simulink model "FINAL100225conmatlab2021"  (R2023a)
settings: Solver=VariableStepAuto  StartTime=0.0  StopTime=100  RelTol=1e-3
libraries: cstblocks x1
settings Model: Creator=cgbri  LastModifiedBy=Maxi
settings RTWCC: GPUComputeCapability=5.0

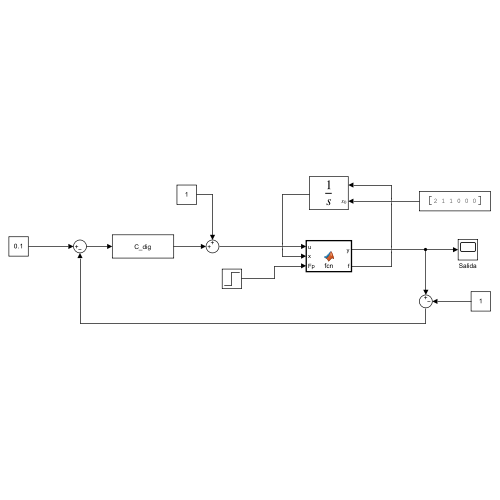
[thumbnail: Simulink's stored preview of the top-level diagram]
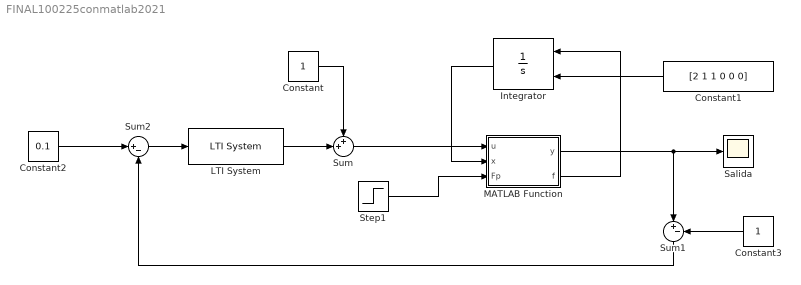
== system FINAL100225conmatlab2021 ==
  Constant : Constant
  Constant1 : Constant  Value=[2 1 1 0 0 0]
  Constant2 : Constant  Value=0.1
  Constant3 : Constant
  Integrator : Integrator  InitialConditionSource=external
  LTI System : cstblocks/LTI System  sys=C_dig  IC=[]
  MATLAB Function : MATLAB Function  TreatAsAtomicUnit=on
  Salida : Scope
  Step1 : Step  After=0  SampleTime=0
  Sum : Sum  Inputs=++|
  Sum1 : Sum  Inputs=|+-
  Sum2 : Sum  Inputs=|+-
  wires:
  Integrator/1 -> MATLAB Function/2(x)
  MATLAB Function/2(f) -> Integrator/1
  Constant1/1 -> Integrator/2
  Step1/1 -> MATLAB Function/3(Fp)
  MATLAB Function/1(y) -> Sum1/1, Salida/1
  Sum/1 -> MATLAB Function/1(u)
  Constant/1 -> Sum/1
  Constant3/1 -> Sum1/2
  Sum1/1 -> Sum2/2
  LTI System/1 -> Sum/2
  Sum2/1 -> LTI System/1
  Constant2/1 -> Sum2/1

== matlab function FINAL100225conmatlab2021/MATLAB Function ==
  data: u input; y output; x input; f output; Fp input
function [y,f] = fcn(u, x, Fp)
    y = x(2);
    f1 = (x(3)-sqrt(x(1)-x(2)))/power(x(1), 2);
    f2 = (sqrt(x(1)-x(2))-sqrt(x(2)) + Fp )/power(x(2), 2);
    f3 = x(4);
    f4 = x(5);
    f5 = x(6);
    f6 = (u - (1/2)*x(6) - (3/2)*x(5) - 2*x(4) - x(3)) * 16;
    f = [f1; f2; f3; f4; f5; f6];
